simulink library "ilcPhaseSwitching_cl"  (R2022a)
settings: Solver=VariableStepAuto  StartTime=0.0  StopTime=10.0  RelTol=1e-3
undefined symbols (not defined in the file or in its folder): hiLvlCtrl
libraries: ctrlSharedLib x1
settings Model: Creator=adabney  LastModifiedBy=adabney

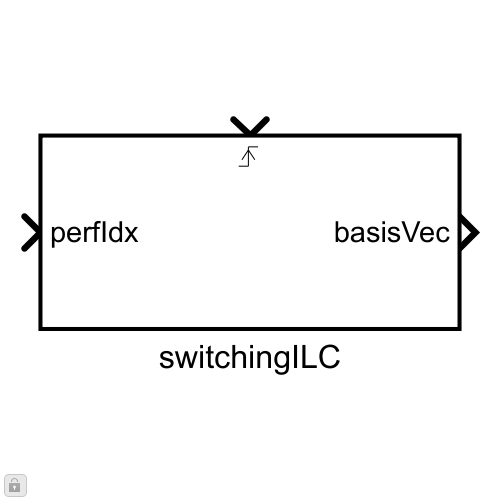
[thumbnail: Simulink's stored preview of the top-level diagram]
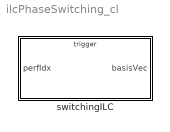
== system ilcPhaseSwitching_cl ==
  switchingILC : Subsystem  mask{hiLvlCtrl=hiLvlCtrl}
      mask prompts: hiLvlCtrl "ILC Controller"
      mask DialogControl ParameterGroupVar Prompt: Controller Settings

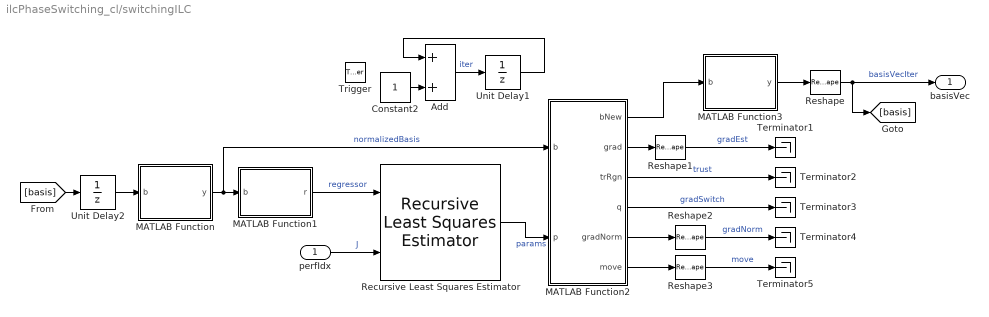
== system ilcPhaseSwitching_cl/switchingILC ==
  perfIdx : Inport  PortDimensions=1
  Trigger : TriggerPort  VariantControl=(inherit)  PortDimensions=1
  Add : Sum
  Constant2 : Constant
  MATLAB Function : MATLAB Function  TreatAsAtomicUnit=on  mask{upperLim=hiLvlCtrl.upperLim(:), lowerLim=hiLvlCtrl.lowerLim(:)}
      mask prompts: upperLim "Upper Limit"; lowerLim "Lower Limit"
  MATLAB Function1 : MATLAB Function  TreatAsAtomicUnit=on
  MATLAB Function2 : MATLAB Function  TreatAsAtomicUnit=on  mask{trust=hiLvlCtrl.trustRegion, amp=hiLvlCtrl.excitationAmp, lrn=hiLvlCtrl.learningGain, switching=hiLvlCtrl.switching.Value, paramDims=hiLvlCtrl.subspaceDims}
      mask prompts: trust "Trust Region"; amp "Persistent Excitation Amplitude"; lrn "Learning Gain"; switching "Switching ILC (1 - yes, 0 - no)"; paramDims "Parameter Space Dimensions"
  MATLAB Function3 : MATLAB Function  TreatAsAtomicUnit=on  mask{upperLim=hiLvlCtrl.upperLim(:), lowerLim=hiLvlCtrl.lowerLim(:)}
      mask prompts: upperLim "Upper Limit"; lowerLim "Lower Limit"
  Recursive Least Squares Estimator : ctrlSharedLib/Recursive Least Squares Estimator  InitialEstimateSource=None  InitialParameterData=2*numel(hiLvlCtrl.initParameters)+1  P0=1e4  InitialRegressors=0  InitialOutputs=0  History=Infinite  WindowLength=200  EstimationMethod=Forgetting Factor  AdaptationParameter=hiLvlCtrl.forgettingFactor.Value  HasTimeVaryingAdaptationParameter=off  NormalizationBias=eps  OutputError=off  OutputP=off  AddEnablePort=off  InputProcessing=Sample-based  Ts=-1
      settings: SourceProductBaseCode=CT,ID
  Reshape{,1..3} (4 alike) : Reshape
  Terminator{1..5} (5 alike) : Terminator
  Unit Delay1 : UnitDelay  SampleTime=-1  HasFrameUpgradeWarning=on
  Unit Delay2 : UnitDelay  InitialCondition=hiLvlCtrl.initParameters  SampleTime=-1  HasFrameUpgradeWarning=on
  basisVec : Outport  InitialOutput=hiLvlCtrl.initParameters
  wires:
  MATLAB Function2/1(bNew) -> MATLAB Function3/1(b)
  MATLAB Function1/1(r) -> Recursive Least Squares Estimator/1  "regressor"
  perfIdx/1 -> Recursive Least Squares Estimator/2  "J"
  MATLAB Function2/2(grad) -> Reshape1/1
  [basis] -> Unit Delay2/1
  Add/1 -> Unit Delay1/1  "iter"
  Unit Delay2/1 -> MATLAB Function/1(b)
  Constant2/1 -> Add/2
  Recursive Least Squares Estimator/1 -> MATLAB Function2/2(p)  "params"
  Reshape/1 -> [basis], basisVec/1  "basisVecIter"
  MATLAB Function/1(y) -> MATLAB Function2/1(b), MATLAB Function1/1(b)  "normalizedBasis"
  MATLAB Function3/1(y) -> Reshape/1
  MATLAB Function2/3(trRgn) -> Terminator2/1  "trust"
  MATLAB Function2/4(q) -> Terminator3/1  "gradSwitch"
  Unit Delay1/1 -> Add/1
  Reshape1/1 -> Terminator1/1  "gradEst"
  MATLAB Function2/6(move) -> Reshape3/1
  MATLAB Function2/5(gradNorm) -> Reshape2/1
  Reshape2/1 -> Terminator4/1  "gradNorm"
  Reshape3/1 -> Terminator5/1  "move"

== matlab function ilcPhaseSwitching_cl/switchingILC/MATLAB Function2 ==
  data: b input; bNew output; p input; lrn parameter; grad output; trust parameter; amp parameter; trRgn output; q output; switching parameter; paramDims parameter; gradNorm output; move output
function [bNew,grad,trRgn,q,gradNorm,move] = fcn(b,p,lrn,trust,amp,switching,paramDims)
b = b(:); %Reshape into column vector
n = numel(b);
p = p(:); % Reshape to column

%Calculate Gradient
grad = p(2:2:end)+2*p(3:2:end).*b(:);

% Calculate Move
move = zeros(n,1); %Initialize the move vector
%
deltaB = lrn(:).*grad;
%

trustRgn = abs(trust(:)./deltaB);
trRgn = min([1;trustRgn]);

m = numel(paramDims);
gradNorm = zeros(1,m);
%Toggle between eILC and seILC
if switching == 0
    %seILC
    %eILC
    move = deltaB*trRgn;
    q = 1;
else
    moveVec = zeros(sum(paramDims),1);
    for i = 1:m
        if i == 1
            moveVec(1:paramDims(i)) = i;
        else
            ind1 = 1+sum(paramDims(1:i-1));
            ind2 = sum(paramDims(1:i));
            moveVec(ind1:ind2) = i;
        end
        gradNorm(i) = norm(grad(moveVec==i));
    end
    % Move in the direction with the largest norm(grad)
    [~,q] = max(gradNorm);
    trRgn = min([1; trustRgn(moveVec==q)]);
    move(moveVec==q) = trRgn*deltaB(moveVec==q);
end

bNew = b + move + amp(:).*trust(:).*(2*rand(n,1)-1);

== matlab function ilcPhaseSwitching_cl/switchingILC/MATLAB Function1 ==
  data: b input; r output
function r = fcn(b)
% Preallocate column vector output
r = ones(1+2*numel(b),1);
% Build matrix of basis params and their squares
b = [b(:) b(:).^2];
% Reshape to column vector and store into output
r(2:end) = reshape(b',[numel(b),1]);

== matlab function ilcPhaseSwitching_cl/switchingILC/MATLAB Function ==
  data: b input; y output; upperLim parameter; lowerLim parameter
function y = fcn(b,upperLim,lowerLim)

y = (b(:)-lowerLim)./(upperLim-lowerLim);

== matlab function ilcPhaseSwitching_cl/switchingILC/MATLAB Function3 ==
  data: b input; y output; upperLim parameter; lowerLim parameter
function y = fcn(b,upperLim,lowerLim)

b(b>1) = 1;
b(b<0) = 0;

y = b(:).*(upperLim-lowerLim)+lowerLim;
if numel(y)>10 && numel(y)~=20
    if y(2) > y(1)/2
        y(2) = y(1)/2;
    end
end
